simulink model "Group_11_ARO_4090_Simulink_Model_HW7_V2"  (R2023b)
settings: Solver=VariableStepAuto  StartTime=0.0  StopTime=30  FixedStep=0.002  RelTol=1e-3  EnableMultiTasking=on
libraries: simulink_extras x8
settings Model: ExtModeTrigDuration=10000  Creator=jtmil  LastModifiedBy=jtmil
settings SolverCC: AlgebraicLoopSolver=TrustRegion  PositivePriorityOrder=on
settings DataIOCC: ReturnWorkspaceOutputs=off
settings OptimizationCC: LifeSpan=inf
settings DebuggingCC: UnconnectedInputMsg=warning  UnconnectedOutputMsg=warning  UnconnectedLineMsg=warning  ArithmeticOperatorsInVariantConditions=warning
settings ModelReferenceCC: EnableRefExpFcnMdlSchedulingChecks=on
settings SFSimCC: SimUseLocalCustomCode=off  CustomCodeUndefinedFunction=UseInterfaceOnly
settings RTWCC: Description=QUARC Win64 Target  SystemTargetFile=quarc_win64.tlc  TemplateMakefile=quarc_default_tmf  RTWUseLocalCustomCode=off
settings CodeAppCC: StateflowObjectComments=on
settings STFCustomTargetCC: TargetPreCompLibLocation=C:\PROGRA~3\QUARC\lib\2016a\win64\release  ConcurrentExecutionCompliant=on  GRTInterface=on  SystemTargetFile=quarc_win64.tlc
settings GRTTargetCC: TargetPreCompLibLocation=C:\PROGRA~3\QUARC\lib\2016a\win64\release  ParMdlRefBuildCompliant=off  CompOptLevelCompliant=off  CombineOutputUpdateFcns=off  MatFileLogging=off  CPPClassGenCompliant=off  GRTInterface=on  UseToolchainInfoCompliant=off  ExtMode=on  ExtModeMexFile=quarc_comm
settings ConfigComp: CovMetricSettings=dswe

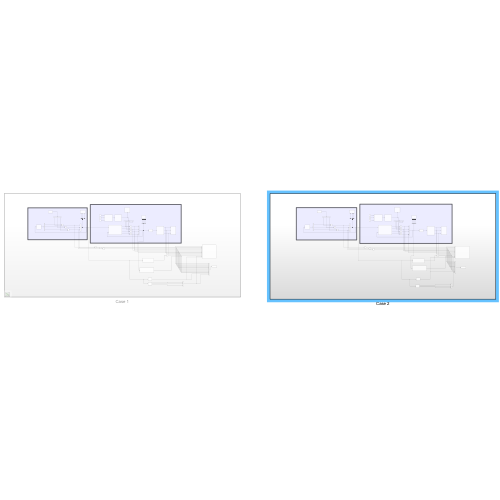
[thumbnail: Simulink's stored preview of the top-level diagram]
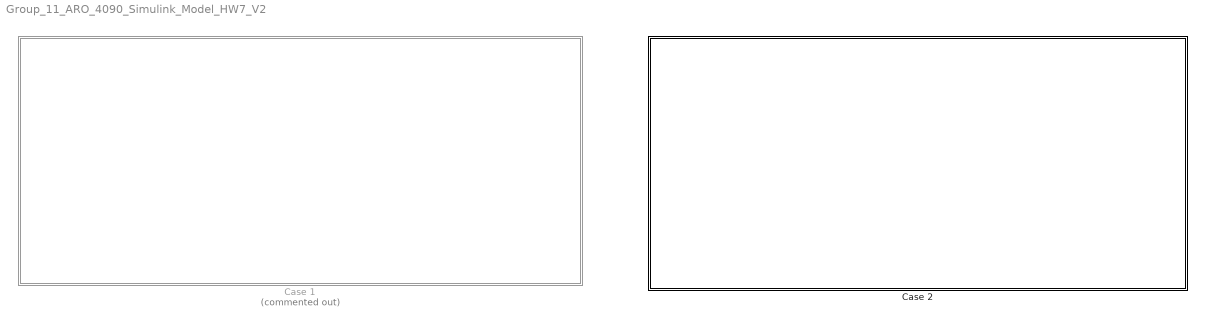
== system Group_11_ARO_4090_Simulink_Model_HW7_V2 ==
  Case 1 : Subsystem  Commented=on
  Case 2 : Subsystem

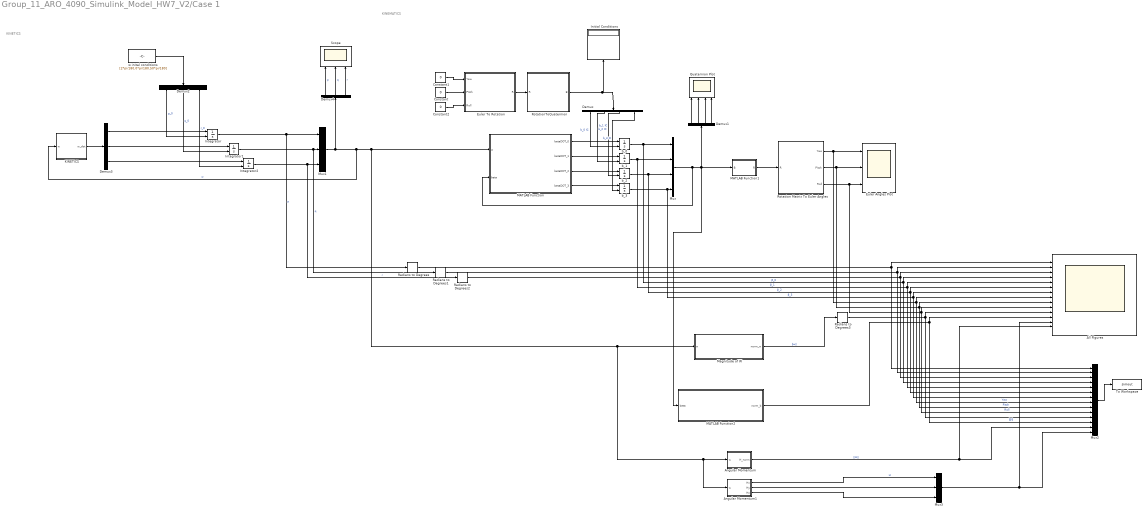
== system Group_11_ARO_4090_Simulink_Model_HW7_V2/Case 1 ==
  note: KINETICS
  note: KINEMATICS
  All FIgures : Scope  NumInputPorts=14
  Angular Momentum : MATLAB Function  TreatAsAtomicUnit=on
  Angular Momentum1 : MATLAB Function  TreatAsAtomicUnit=on
  Constant : Constant  Value=0
  Constant1 : Constant  Value=0
  Constant2 : Constant  Value=0
  Demux : Demux
  Demux1 : Demux
  Demux2 : Demux  Outputs=3
  Demux3 : Demux  Outputs=3
  Demux4 : Demux  Outputs=3
  Euler Angles Plot : Scope  NumInputPorts=3
  Euler To Rotation : MATLAB Function  TreatAsAtomicUnit=on
  Initial Conditions : Display
  Integrator : Integrator  InitialConditionSource=external
  Integrator1 : Integrator  InitialConditionSource=external
  Integrator2 : Integrator  InitialConditionSource=external
  KINETICS : MATLAB Function  TreatAsAtomicUnit=on
  MATLAB Function : MATLAB Function  TreatAsAtomicUnit=on
  MATLAB Function1 : MATLAB Function  TreatAsAtomicUnit=on
  MATLAB Function2 : MATLAB Function  TreatAsAtomicUnit=on
  Magnitude of W : MATLAB Function  TreatAsAtomicUnit=on
  Mux : Mux
  Mux1 : Mux  Inputs=3
  Mux2 : Mux  Inputs=14
  Mux3 : Mux  Inputs=3
  Quaternion Plot : Scope  NumInputPorts=4
  Radians to Degrees{,1..3} (4 alike) : simulink_extras/Transformations/Radians to Degrees
  Rotation Matrix To Euler Angles : MATLAB Function  TreatAsAtomicUnit=on
  RotationToQuaternion : MATLAB Function  TreatAsAtomicUnit=on
  Scope : Scope  NumInputPorts=3
  To Workspace : ToWorkspace  VariableName=simout  SaveFormat=Timeseries  SampleTime=-1
  b_{0..3} (4 alike) : Integrator  InitialConditionSource=external
  w inital conditions : Constant  Value=[2*pi/180,0*pi/180,50*pi/180]
  wires:
  Demux1/4 -> Quaternion Plot/4
  Constant/1 -> Euler To Rotation/2(Pitch)
  Rotation Matrix To Euler Angles/2(Pitch) -> Mux2/9, All FIgures/9, Euler Angles Plot/2  "Pitch"
  Integrator1/1 -> Radians to Degrees1/1, Mux1/2  "q"
  b_2/1 -> Mux/3, Mux2/6, All FIgures/6  "β_2"
  b_0/1 -> Mux/1, Mux2/4, All FIgures/4  "β_0"
  Demux1/1 -> Quaternion Plot/1
  Magnitude of W/1(norm_w) -> Radians to Degrees3/1  "∥ω∥"
  Integrator/1 -> Radians to Degrees/1, Mux1/1  "p"
  MATLAB Function2/1(norm_b) -> Mux2/12, All FIgures/12  "∥β∥"
  Demux4/2 -> Scope/2  "q"
  MATLAB Function/3(betaDOT_2) -> b_2/1
  RotationToQuaternion/1(B) -> Initial Conditions/1, Demux/1
  Constant1/1 -> Euler To Rotation/1(Yaw)
  Demux/4 -> b_3/2  "b_3 IC"
  MATLAB Function/1(betaDOT_0) -> b_0/1
  Mux1/1 -> Angular Momentum1/1(w), Angular Momentum/1(w), Magnitude of W/1(w), MATLAB Function/1(w), KINETICS/1(w), Demux4/1  "w"
  Demux4/1 -> Scope/1  "p"
  Demux4/3 -> Scope/3  "r"
  Rotation Matrix To Euler Angles/1(Yaw) -> Euler Angles Plot/1, Mux2/8, All FIgures/8  "Yaw"
  b_1/1 -> Mux/2, Mux2/5, All FIgures/5  "β_1"
  Demux2/2 -> Integrator1/2  "q_0"
  b_3/1 -> Mux2/7, All FIgures/7, Mux/4  "β_3"
  Rotation Matrix To Euler Angles/3(Roll) -> Mux2/10, All FIgures/10, Euler Angles Plot/3  "Roll"
  Radians to Degrees/1 -> All FIgures/1, Mux2/1
  Radians to Degrees2/1 -> Mux2/3, All FIgures/3
  Radians to Degrees1/1 -> Mux2/2, All FIgures/2
  Euler To Rotation/1(R) -> RotationToQuaternion/1(R)
  Radians to Degrees3/1 -> Mux2/11, All FIgures/11
  Integrator2/1 -> Radians to Degrees2/1, Mux1/3  "r"
  Mux2/1 -> To Workspace/1
  Demux1/3 -> Quaternion Plot/3
  MATLAB Function/4(betaDOT_3) -> b_3/1
  Demux1/2 -> Quaternion Plot/2
  Mux/1 -> MATLAB Function/2(beta), Demux1/1, MATLAB Function2/1(beta), MATLAB Function1/1(B)
  Demux3/3 -> Integrator2/1
  MATLAB Function1/1(R) -> Rotation Matrix To Euler Angles/1(R)
  Demux2/1 -> Integrator/2  "p_0"
  MATLAB Function/2(betaDOT_1) -> b_1/1
  Demux2/3 -> Integrator2/2  "r_0"
  Demux3/1 -> Integrator/1
  Demux/2 -> b_1/2  "b_1 IC"
  Demux/3 -> b_2/2  "b_2 IC"
  w inital conditions/1 -> Demux2/1
  Demux/1 -> b_0/2  "b_0 IC"
  KINETICS/1(w_dot) -> Demux3/1
  Demux3/2 -> Integrator1/1
  Constant2/1 -> Euler To Rotation/3(Roll)
  Angular Momentum/1(H_norm) -> All FIgures/14, Mux2/13  "||H||"
  Angular Momentum1/1(Hx) -> Mux3/1  "H"
  Angular Momentum1/2(Hy) -> Mux3/2
  Angular Momentum1/3(Hz) -> Mux3/3
  Mux3/1 -> All FIgures/13, Mux2/14

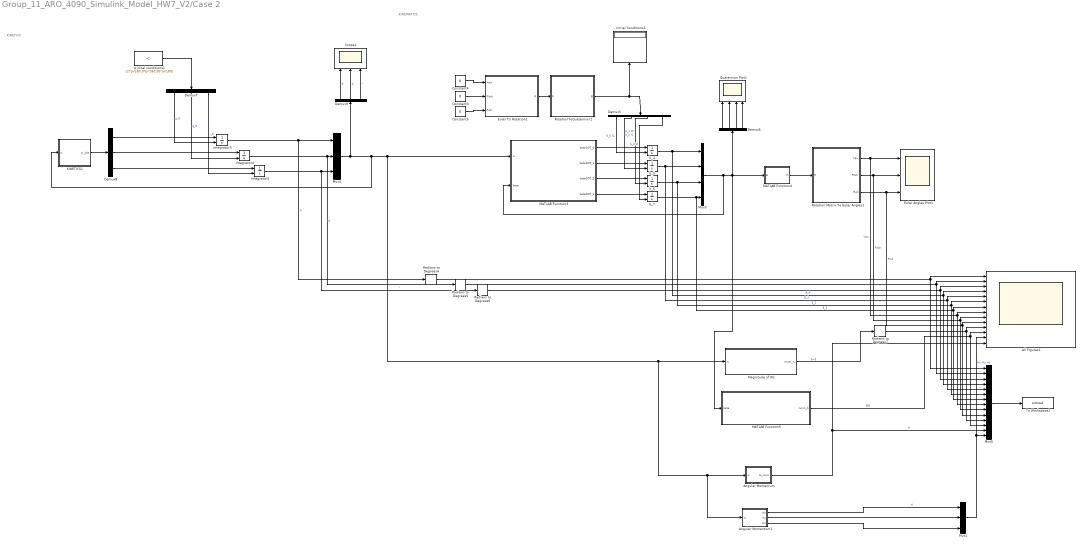
== system Group_11_ARO_4090_Simulink_Model_HW7_V2/Case 2 ==
  note: KINETICS
  note: KINEMATICS
  All FIgures1 : Scope  NumInputPorts=14
  Angular Momentum : MATLAB Function  TreatAsAtomicUnit=on
  Angular Momentum1 : MATLAB Function  TreatAsAtomicUnit=on
  Constant3 : Constant  Value=0
  Constant4 : Constant  Value=0
  Constant5 : Constant  Value=0
  Demux5 : Demux
  Demux6 : Demux
  Demux7 : Demux  Outputs=3
  Demux8 : Demux  Outputs=3
  Demux9 : Demux  Outputs=3
  Euler Angles Plot1 : Scope  NumInputPorts=3
  Euler To Rotation1 : MATLAB Function  TreatAsAtomicUnit=on
  Initial Conditions1 : Display
  Integrator3 : Integrator  InitialConditionSource=external
  Integrator4 : Integrator  InitialConditionSource=external
  Integrator5 : Integrator  InitialConditionSource=external
  KINETICS1 : MATLAB Function  TreatAsAtomicUnit=on
  MATLAB Function3 : MATLAB Function  TreatAsAtomicUnit=on
  MATLAB Function4 : MATLAB Function  TreatAsAtomicUnit=on
  MATLAB Function5 : MATLAB Function  TreatAsAtomicUnit=on
  Magnitude of W1 : MATLAB Function  TreatAsAtomicUnit=on
  Mux1 : Mux  Inputs=3
  Mux3 : Mux
  Mux4 : Mux  Inputs=3
  Mux5 : Mux  Inputs=14
  Quaternion Plot1 : Scope  NumInputPorts=4
  Radians to Degrees{4..7} (4 alike) : simulink_extras/Transformations/Radians to Degrees
  Rotation Matrix To Euler Angles1 : MATLAB Function  TreatAsAtomicUnit=on
  RotationToQuaternion1 : MATLAB Function  TreatAsAtomicUnit=on
  Scope1 : Scope  NumInputPorts=3
  To Workspace1 : ToWorkspace  VariableName=simout  SaveFormat=Timeseries  SampleTime=-1
  b_{4..7} (4 alike) : Integrator  InitialConditionSource=external
  w inital conditions1 : Constant  Value=[2*pi/180,0*pi/180,50*pi/180]
  wires:
  MATLAB Function3/1(betaDOT_0) -> b_4/1
  Radians to Degrees5/1 -> Mux5/2, All FIgures1/2
  Demux7/1 -> Integrator3/2  "p_0"
  b_6/1 -> Mux3/3, Mux5/6, All FIgures1/6  "β_2"
  MATLAB Function3/4(betaDOT_3) -> b_7/1
  MATLAB Function3/2(betaDOT_1) -> b_5/1
  Rotation Matrix To Euler Angles1/3(Roll) -> Mux5/10, All FIgures1/10, Euler Angles Plot1/3  "Roll"
  Demux5/4 -> b_7/2  "b_3 IC"
  Integrator5/1 -> Radians to Degrees6/1, Mux4/3  "r"
  Demux6/2 -> Quaternion Plot1/2
  Constant4/1 -> Euler To Rotation1/1(Yaw)
  Demux5/1 -> b_4/2  "b_0 IC"
  Mux3/1 -> MATLAB Function3/2(beta), Demux6/1, MATLAB Function5/1(beta), MATLAB Function4/1(B)
  RotationToQuaternion1/1(B) -> Initial Conditions1/1, Demux5/1
  Integrator3/1 -> Radians to Degrees4/1, Mux4/1  "p"
  b_4/1 -> Mux3/1, Mux5/4, All FIgures1/4  "β_0"
  Demux6/3 -> Quaternion Plot1/3
  MATLAB Function5/1(norm_b) -> Mux5/12, All FIgures1/12  "∥β∥"
  Radians to Degrees4/1 -> All FIgures1/1, Mux5/1
  Demux8/2 -> Integrator4/1
  Demux6/1 -> Quaternion Plot1/1
  Mux5/1 -> To Workspace1/1
  Demux8/3 -> Integrator5/1
  KINETICS1/1(w_dot) -> Demux8/1
  Constant5/1 -> Euler To Rotation1/3(Roll)
  Integrator4/1 -> Radians to Degrees5/1, Mux4/2  "q"
  Rotation Matrix To Euler Angles1/2(Pitch) -> Mux5/9, All FIgures1/9, Euler Angles Plot1/2  "Pitch"
  b_7/1 -> Mux5/7, All FIgures1/7, Mux3/4  "β_3"
  Demux5/3 -> b_6/2  "b_2 IC"
  w inital conditions1/1 -> Demux7/1
  Mux4/1 -> Angular Momentum1/1(w), Angular Momentum/1(w), Magnitude of W1/1(w), MATLAB Function3/1(w), KINETICS1/1(w), Demux9/1
  Demux6/4 -> Quaternion Plot1/4
  Demux7/3 -> Integrator5/2  "r_0"
  b_5/1 -> Mux3/2, Mux5/5, All FIgures1/5  "β_1"
  Radians to Degrees6/1 -> Mux5/3, All FIgures1/3
  Demux5/2 -> b_5/2  "b_1 IC"
  Radians to Degrees7/1 -> Mux5/11, All FIgures1/11
  Magnitude of W1/1(norm_w) -> Radians to Degrees7/1  "∥ω∥"
  Demux8/1 -> Integrator3/1
  Euler To Rotation1/1(R) -> RotationToQuaternion1/1(R)
  MATLAB Function4/1(R) -> Rotation Matrix To Euler Angles1/1(R)
  Rotation Matrix To Euler Angles1/1(Yaw) -> Euler Angles Plot1/1, Mux5/8, All FIgures1/8  "Yaw"
  Demux9/2 -> Scope1/2  "q"
  Demux7/2 -> Integrator4/2  "q_0"
  Demux9/3 -> Scope1/3  "r"
  MATLAB Function3/3(betaDOT_2) -> b_6/1
  Demux9/1 -> Scope1/1  "p"
  Constant3/1 -> Euler To Rotation1/2(Pitch)
  Angular Momentum/1(H_norm) -> Mux5/13, All FIgures1/14  "H"
  Angular Momentum1/3(Hz) -> Mux1/3
  Angular Momentum1/2(Hy) -> Mux1/2
  Angular Momentum1/1(Hx) -> Mux1/1  "H"
  Mux1/1 -> All FIgures1/13, Mux5/14  "Hx Hy Hz"

== matlab function Group_11_ARO_4090_Simulink_Model_HW7_V2/Case 2/MATLAB Function4 ==
  data: B input; R output
function R  = QuaterToRot(B)


R = [B(1)^2 + B(2)^2 - B(3)^2 - B(4)^2, 2*B(2)*B(3) + 2*B(1)*B(4), 2*B(2)*B(4) - 2*B(1)*B(3);
     2*B(2)*B(3) - 2*B(1)*B(4), B(1)^2 - B(2)^2 + B(3)^2 - B(4)^2, 2*B(3)*B(4) + 2*B(1)*B(2);
     2*B(2)*B(4) + 2*B(1)*B(3), 2*B(3)*B(4) - 2*B(1)*B(2), B(1)^2 - B(2)^2 - B(3)^2 + B(4)^2];



end

== matlab function Group_11_ARO_4090_Simulink_Model_HW7_V2/Case 2/MATLAB Function5 ==
  data: beta input; norm_b output
function norm_b = Magnitude(beta)

norm_b = norm(beta)
end

== matlab function Group_11_ARO_4090_Simulink_Model_HW7_V2/Case 2/Magnitude of W1 ==
  data: w input; norm_w output
function norm_w = Magnitude(w)
norm_w = norm(w)
end

== matlab function Group_11_ARO_4090_Simulink_Model_HW7_V2/Case 2/Rotation Matrix To Euler Angles1 ==
  data: Yaw output; Pitch output; R input; Roll output
function [Yaw,Pitch,Roll] = RotToEuler(R)

Yaw = atan2d(R(1,2) , R(1,1)) % Yaw
Pitch = asind(-R(1,3))        % Pitch
Roll = atan2d(R(2,3),R(3,3))   % Roll

if Yaw<0
        Yaw=mod(Yaw+360,360);
    end

end

== matlab function Group_11_ARO_4090_Simulink_Model_HW7_V2/Case 2/RotationToQuaternion1 ==
  data: R input; B output
function B = RotToQuaternion(R)

B_0_check = (1/4)*(1 + R(1,1) + R(2,2) + R(3,3));
B_1_check = (1/4)*(1 + R(1,1) - R(2,2) - R(3,3));
B_2_check = (1/4)*(1 + R(2,2) - R(1,1) - R(3,3));
B_3_check = (1/4)*(1 + R(3,3) - R(1,1) - R(2,2));

B_check = [B_0_check ; B_1_check ; B_2_check ; B_3_check];

B_max = max(B_check);

% Initialize variables to ensure they are defined
B_0 = 0;
B_1 = 0;
B_2 = 0;
B_3 = 0;

if B_max == B_0_check % B_0 is max
    B_0 = sqrt(B_0_check);
    B_1 = (1/(4*B_0))*(R(2,3) - R(3,2));
    B_2 = (1/(4*B_0))*(R(3,1) - R(1,3));
    B_3 = (1/(4*B_0))*(R(1,2) - R(2,1));
elseif B_max == B_1_check % B_1 is max
    B_1 = sqrt(B_1_check);
    B_0 = (1/(4*B_1))*(R(2,3) - R(3,2));
    B_2 = (1/(4*B_1))*(R(1,2) - R(2,1));
    B_3 = (1/(4*B_1))*(R(3,1) - R(1,3));
elseif B_max == B_2_check % B_2 is max
    B_2 = sqrt(B_2_check);
    B_0 = (1/(4*B_2))*(R(3,1) - R(1,3));
    B_1 = (1/(4*B_2))*(R(1,2) + R(2,1));
    B_3 = (1/(4*B_2))*(R(2,3) + R(3,2));
elseif B_max == B_3_check % B_3 is max
    B_3 = sqrt(B_3_check);
    B_0 = (1/(4*B_3))*(R(1,2) - R(2,1));
    B_1 = (1/(4*B_3))*(R(3,1) + R(1,3));
    B_2 = (1/(4*B_3))*(R(2,3) + R(3,2));
end

B = [B_0 ; B_1 ; B_2 ; B_3];

if any(B < 0)
    B = -1*B;
end

end

== matlab function Group_11_ARO_4090_Simulink_Model_HW7_V2/Case 1/Angular Momentum ==
  data: w input; H_norm output
function H_norm = fcn(w)

M = (10^-2)*[0 ; 0 ; 0];

a = 0.01 ; e = a ; b = 0.03 ; c = 0.005 ; d = 0.06;

rho = 1000;

num = (b*c)*(a+b);
den = 2*(a*d + b*c);
R_x = [ 0 , -(a/2) - num/den , 0 ; (a/2) + num/den , 0  , 0 ; 0 , 0 , 0];
I_B_o = zeros(3, 3); 
I_B_o(1,1) = (rho/12)*(a*d*e*(4*a^2 + d^2) + b*c*e*(4*b^2 +c^2 + 12*a^2 + 12*a*b));
I_B_o(2,2) = (rho/12)*(a*d*e*(4*a^2 + e^2) + b*c*e*(4*b^2 +e^2 + 12*a^2 + 12*a*b));
I_B_o(3,3) = (rho/12)*(a*e*d*(e^2 + d^2) + b*c*e*(e^2 + c^2));


R_x_sq = R_x * R_x;
mass = rho*(a*d*e + b*c*e)

I_B = I_B_o + mass.*R_x_sq  

H = I_B*w;

H_norm= norm(H);

== matlab function Group_11_ARO_4090_Simulink_Model_HW7_V2/Case 2/Angular Momentum ==
  data: w input; H_norm output
function H_norm = fcn(w)

M = (10^-2)*[0 ; 0 ; 0];

a = 0.01 ; e = a ; b = 0.05 ; c = 0.005 ; d = 0.06;

rho = 1000;

num = (b*c)*(a+b);
den = 2*(a*d + b*c);
R_x = [ 0 , -(a/2) - num/den , 0 ; (a/2) + num/den , 0  , 0 ; 0 , 0 , 0];
I_B_o = zeros(3, 3); 
I_B_o(1,1) = (rho/12)*(a*d*e*(4*a^2 + d^2) + b*c*e*(4*b^2 +c^2 + 12*a^2 + 12*a*b));
I_B_o(2,2) = (rho/12)*(a*d*e*(4*a^2 + e^2) + b*c*e*(4*b^2 +e^2 + 12*a^2 + 12*a*b));
I_B_o(3,3) = (rho/12)*(a*e*d*(e^2 + d^2) + b*c*e*(e^2 + c^2));


R_x_sq = R_x * R_x;
mass = rho*(a*d*e + b*c*e)

I_B = I_B_o + mass.*R_x_sq  

H = I_B*w;

H_norm= norm(H);

== matlab function Group_11_ARO_4090_Simulink_Model_HW7_V2/Case 1/Angular Momentum1 ==
  data: w input; Hx output; Hy output; Hz output
function [Hx,Hy,Hz] = fcn(w)

M = (10^-2)*[0 ; 0 ; 0];

a = 0.01 ; e = a ; b = 0.03 ; c = 0.005 ; d = 0.06;

rho = 1000;

num = (b*c)*(a+b);
den = 2*(a*d + b*c);
R_x = [ 0 , -(a/2) - num/den , 0 ; (a/2) + num/den , 0  , 0 ; 0 , 0 , 0];
I_B_o = zeros(3, 3); 
I_B_o(1,1) = (rho/12)*(a*d*e*(4*a^2 + d^2) + b*c*e*(4*b^2 +c^2 + 12*a^2 + 12*a*b));
I_B_o(2,2) = (rho/12)*(a*d*e*(4*a^2 + e^2) + b*c*e*(4*b^2 +e^2 + 12*a^2 + 12*a*b));
I_B_o(3,3) = (rho/12)*(a*e*d*(e^2 + d^2) + b*c*e*(e^2 + c^2));


R_x_sq = R_x * R_x;
mass = rho*(a*d*e + b*c*e)

I_B = I_B_o + mass.*R_x_sq  

H = I_B*w;

Hx = H(1)
Hy = H(2)
Hz = H(3)

== matlab function Group_11_ARO_4090_Simulink_Model_HW7_V2/Case 1/Magnitude of W ==
  data: w input; norm_w output
function norm_w = Magnitude(w)
norm_w = norm(w)
end

== matlab function Group_11_ARO_4090_Simulink_Model_HW7_V2/Case 2/Angular Momentum1 ==
  data: w input; Hx output; Hy output; Hz output
function [Hx,Hy,Hz] = fcn(w)

M = (10^-2)*[0 ; 0 ; 0];

a = 0.01 ; e = a ; b = 0.03 ; c = 0.005 ; d = 0.06;

rho = 1000;

num = (b*c)*(a+b);
den = 2*(a*d + b*c);
R_x = [ 0 , -(a/2) - num/den , 0 ; (a/2) + num/den , 0  , 0 ; 0 , 0 , 0];
I_B_o = zeros(3, 3); 
I_B_o(1,1) = (rho/12)*(a*d*e*(4*a^2 + d^2) + b*c*e*(4*b^2 +c^2 + 12*a^2 + 12*a*b));
I_B_o(2,2) = (rho/12)*(a*d*e*(4*a^2 + e^2) + b*c*e*(4*b^2 +e^2 + 12*a^2 + 12*a*b));
I_B_o(3,3) = (rho/12)*(a*e*d*(e^2 + d^2) + b*c*e*(e^2 + c^2));


R_x_sq = R_x * R_x;
mass = rho*(a*d*e + b*c*e)

I_B = I_B_o + mass.*R_x_sq  

H = I_B*w;

Hx = H(1)
Hy = H(2)
Hz = H(3)

== matlab function Group_11_ARO_4090_Simulink_Model_HW7_V2/Case 1/MATLAB Function ==
  data: w input; betaDOT_0 output; beta input; betaDOT_1 output; betaDOT_2 output; betaDOT_3 output
function [betaDOT_0 , betaDOT_1 , betaDOT_2 , betaDOT_3]= KINEMATICS(w , beta)


B_Beta = [-beta(2) -beta(3) -beta(4) ;
        beta(1) -beta(4) beta(3);
        beta(4) beta(1) -beta(2);
        -beta(3) beta(2) beta(1);]

beta_dot = 0.5*B_Beta*w

betaDOT_0 = beta_dot(1)
betaDOT_1 = beta_dot(2)
betaDOT_2 = beta_dot(3)
betaDOT_3 = beta_dot(4)



end

== matlab function Group_11_ARO_4090_Simulink_Model_HW7_V2/Case 1/Euler To Rotation ==
  data: Yaw input; R output; Pitch input; Roll input
function R  = EulerToRot(Yaw,Pitch, Roll)

R1 = [ 1 0 0  ; 0 cosd(Roll) sind(Roll) ; 0 -sind(Roll) cosd(Roll)];
R2 = [cosd(Pitch) 0 -sind(Pitch); 0 1 0; sind(Pitch) 0 cosd(Pitch)];
R3 = [ cosd(Yaw) sind(Yaw) 0 ; -sind(Yaw) cosd(Yaw) 0 ; 0 0 1];

R = R1*R2*R3

end

== matlab function Group_11_ARO_4090_Simulink_Model_HW7_V2/Case 1/Rotation Matrix To Euler Angles ==
  data: Yaw output; Pitch output; R input; Roll output
function [Yaw,Pitch,Roll] = RotToEuler(R)

Yaw = atan2d(R(1,2) , R(1,1)) % Yaw
Pitch = asind(-R(1,3))        % Pitch
Roll = atan2d(R(2,3),R(3,3))   % Roll

if Yaw<0
        Yaw=mod(Yaw+360,360);
    end

end

== matlab function Group_11_ARO_4090_Simulink_Model_HW7_V2/Case 1/KINETICS ==
  data: w_dot output size=[3,1]; w input size=[3,1]
function w_dot = KINETICS(w)



% M = (10^-2)*[-6*w(1) ; 0 ; -5*w(3)];
M = (10^-2)*[0 ; 0 ; 0];

a = 0.01 ; e = a ; b = 0.03 ; c = 0.005 ; d = 0.06;

rho = 1000;

num = (b*c)*(a+b);
den = 2*(a*d + b*c);
R_x = [ 0 , -(a/2) - num/den , 0 ; (a/2) + num/den , 0  , 0 ; 0 , 0 , 0];
I_B_o = zeros(3, 3); 
I_B_o(1,1) = (rho/12)*(a*d*e*(4*a^2 + d^2) + b*c*e*(4*b^2 +c^2 + 12*a^2 + 12*a*b));
I_B_o(2,2) = (rho/12)*(a*d*e*(4*a^2 + e^2) + b*c*e*(4*b^2 +e^2 + 12*a^2 + 12*a*b));
I_B_o(3,3) = (rho/12)*(a*e*d*(e^2 + d^2) + b*c*e*(e^2 + c^2));


R_x_sq = R_x * R_x;
mass = rho*(a*d*e + b*c*e)

I_B = I_B_o + mass.*R_x_sq  


w_skew = [ 0,     -w(3),  w(2);
           w(3),  0,     -w(1);
           -w(2),  w(1),  0];

w_dot = inv(I_B) * (M - w_skew*I_B*w)


end

== matlab function Group_11_ARO_4090_Simulink_Model_HW7_V2/Case 1/RotationToQuaternion ==
  data: R input; B output
function B = RotToQuaternion(R)

B_0_check = (1/4)*(1 + R(1,1) + R(2,2) + R(3,3));
B_1_check = (1/4)*(1 + R(1,1) - R(2,2) - R(3,3));
B_2_check = (1/4)*(1 + R(2,2) - R(1,1) - R(3,3));
B_3_check = (1/4)*(1 + R(3,3) - R(1,1) - R(2,2));

B_check = [B_0_check ; B_1_check ; B_2_check ; B_3_check];

B_max = max(B_check);

% Initialize variables to ensure they are defined
B_0 = 0;
B_1 = 0;
B_2 = 0;
B_3 = 0;

if B_max == B_0_check % B_0 is max
    B_0 = sqrt(B_0_check);
    B_1 = (1/(4*B_0))*(R(2,3) - R(3,2));
    B_2 = (1/(4*B_0))*(R(3,1) - R(1,3));
    B_3 = (1/(4*B_0))*(R(1,2) - R(2,1));
elseif B_max == B_1_check % B_1 is max
    B_1 = sqrt(B_1_check);
    B_0 = (1/(4*B_1))*(R(2,3) - R(3,2));
    B_2 = (1/(4*B_1))*(R(1,2) - R(2,1));
    B_3 = (1/(4*B_1))*(R(3,1) - R(1,3));
elseif B_max == B_2_check % B_2 is max
    B_2 = sqrt(B_2_check);
    B_0 = (1/(4*B_2))*(R(3,1) - R(1,3));
    B_1 = (1/(4*B_2))*(R(1,2) + R(2,1));
    B_3 = (1/(4*B_2))*(R(2,3) + R(3,2));
elseif B_max == B_3_check % B_3 is max
    B_3 = sqrt(B_3_check);
    B_0 = (1/(4*B_3))*(R(1,2) - R(2,1));
    B_1 = (1/(4*B_3))*(R(3,1) + R(1,3));
    B_2 = (1/(4*B_3))*(R(2,3) + R(3,2));
end

B = [B_0 ; B_1 ; B_2 ; B_3];

if any(B < 0)
    B = -1*B;
end

end

== matlab function Group_11_ARO_4090_Simulink_Model_HW7_V2/Case 1/MATLAB Function1 ==
  data: B input; R output
function R  = QuaterToRot(B)


R = [B(1)^2 + B(2)^2 - B(3)^2 - B(4)^2, 2*B(2)*B(3) + 2*B(1)*B(4), 2*B(2)*B(4) - 2*B(1)*B(3);
     2*B(2)*B(3) - 2*B(1)*B(4), B(1)^2 - B(2)^2 + B(3)^2 - B(4)^2, 2*B(3)*B(4) + 2*B(1)*B(2);
     2*B(2)*B(4) + 2*B(1)*B(3), 2*B(3)*B(4) - 2*B(1)*B(2), B(1)^2 - B(2)^2 - B(3)^2 + B(4)^2];



end

== matlab function Group_11_ARO_4090_Simulink_Model_HW7_V2/Case 1/MATLAB Function2 ==
  data: beta input; norm_b output
function norm_b = Magnitude(beta)

norm_b = norm(beta)
end

== matlab function Group_11_ARO_4090_Simulink_Model_HW7_V2/Case 2/Euler To Rotation1 ==
  data: Yaw input; R output; Pitch input; Roll input
function R  = EulerToRot(Yaw,Pitch, Roll)

R1 = [ 1 0 0  ; 0 cosd(Roll) sind(Roll) ; 0 -sind(Roll) cosd(Roll)];
R2 = [cosd(Pitch) 0 -sind(Pitch); 0 1 0; sind(Pitch) 0 cosd(Pitch)];
R3 = [ cosd(Yaw) sind(Yaw) 0 ; -sind(Yaw) cosd(Yaw) 0 ; 0 0 1];

R = R1*R2*R3

end

== matlab function Group_11_ARO_4090_Simulink_Model_HW7_V2/Case 2/KINETICS1 ==
  data: w_dot output size=[3,1]; w input size=[3,1]
function w_dot = KINETICS(w)



% M = (10^-2)*[-6*w(1) ; 0 ; -5*w(3)];
M = (10^-2)*[0 ; 0 ; 0];

a = 0.01 ; e = a ; b = 0.05 ; c = 0.005 ; d = 0.06;

rho = 1000;

num = (b*c)*(a+b);
den = 2*(a*d + b*c);
R_x = [ 0 , -(a/2) - num/den , 0 ; (a/2) + num/den , 0  , 0 ; 0 , 0 , 0];
I_B_o = zeros(3, 3); 
I_B_o(1,1) = (rho/12)*(a*d*e*(4*a^2 + d^2) + b*c*e*(4*b^2 +c^2 + 12*a^2 + 12*a*b));
I_B_o(2,2) = (rho/12)*(a*d*e*(4*a^2 + e^2) + b*c*e*(4*b^2 +e^2 + 12*a^2 + 12*a*b));
I_B_o(3,3) = (rho/12)*(a*e*d*(e^2 + d^2) + b*c*e*(e^2 + c^2));


R_x_sq = R_x * R_x;
mass = rho*(a*d*e + b*c*e)

I_B = I_B_o + mass.*R_x_sq  


w_skew = [ 0,     -w(3),  w(2);
           w(3),  0,     -w(1);
           -w(2),  w(1),  0];

w_dot = inv(I_B) * (M - w_skew*I_B*w)


end

== matlab function Group_11_ARO_4090_Simulink_Model_HW7_V2/Case 2/MATLAB Function3 ==
  data: w input; betaDOT_0 output; beta input; betaDOT_1 output; betaDOT_2 output; betaDOT_3 output
function [betaDOT_0 , betaDOT_1 , betaDOT_2 , betaDOT_3]= KINEMATICS(w , beta)


B_Beta = [-beta(2) -beta(3) -beta(4) ;
        beta(1) -beta(4) beta(3);
        beta(4) beta(1) -beta(2);
        -beta(3) beta(2) beta(1);]

beta_dot = 0.5*B_Beta*w

betaDOT_0 = beta_dot(1)
betaDOT_1 = beta_dot(2)
betaDOT_2 = beta_dot(3)
betaDOT_3 = beta_dot(4)



end
